simulink model "sim_rx160_two"  (R2020a)
settings: Solver=FixedStepAuto  StartTime=0.0  StopTime=25.0  FixedStep=0.0001  RelTol=1e-3
values from neighbouring files (symbols this model uses):
  cnc_comp = 1    [run_sim_two.m]
  ctc_switch = 0    [run_sim_two.m]
  ctrl_at_end = 1    [run_sim_two.m]
  ctrl_space = 1    [run_sim_two.m]
  ea_set = 4    [run_sim_two.m]
  ea_set2 = 4    [run_sim_two.m]
  ee_att_1 = 3    [run_sim_two.m]
  ee_att_2 = 4    [run_sim_two.m]
  f_des = [0;60;0;0;0;0]    [run_sim_two.m]
  force_ffwd = 1    [run_sim_two.m]
  fp = [p_ef;r_ef]    [run_sim_two.m]
  fp2 = [p_ef2;r_ef2]    [run_sim_two.m]
  frc_comp = 0    [run_sim_two.m]
  grv_comp = 1    [run_sim_two.m]
  ip = [p_ei;r_ei]    [run_sim_two.m]
  ip2 = [p_ei2;r_ei2]    [run_sim_two.m]
  K = 15000    [run_sim_two.m]
  Kc = 0.005    [run_sim_two.m]
  Kd = [10;10;10;7;7;7]    [run_sim_two.m]
  Kdf = [0;10;0;0;0;0]    [run_sim_two.m]
  Ki = [20;20;20;5;5;5]    [run_sim_two.m]
  Kif = [0;0.05;0;0;0;0]    [run_sim_two.m]
  Km = [1;1;1;1;1;1]    [run_sim_two.m]
  Kp = [2550;2250;2750;1150;850;650]    [run_sim_two.m]
  Kpf = [0;3;0;0;0;0]    [run_sim_two.m]
  orn_at_norm = 1    [run_sim_two.m]
  prdc_frc = 0    [run_sim_two.m]
  q_posIni = qi    [run_sim_two.m]
  robot_model_1 = 2    [run_sim_two.m]
  robot_model_2 = 3    [run_sim_two.m]
  rpt_num = 1    [run_sim_two.m]
  rpt_num2 = 10    [run_sim_two.m]
  Sf_diag = [0;1;0;0;0;0]    [run_sim_two.m]
  spr_comp = 1    [run_sim_two.m]
  switch_val = 30    [run_sim_two.m]
  Sx_diag = [1;0;1;1;1;1]    [run_sim_two.m]
  tf2 = rpt_num2 * period2    (= 30)    [run_sim_two.m]
  trj_profile = 3    [run_sim_two.m]
  trj_profile2 = 3    [run_sim_two.m]
  trj_space = 1    [run_sim_two.m]
  trj_space2 = 1    [run_sim_two.m]
  trj_type = 2    [run_sim_two.m]
  trj_type2 = 1    [run_sim_two.m]
undefined symbols (not defined in the file or in its folder): delta
libraries: simulink x2, vrlib x1
(part 1 of 4)
settings Model: Creator=Mertcan  LastModifiedBy=Mertcan

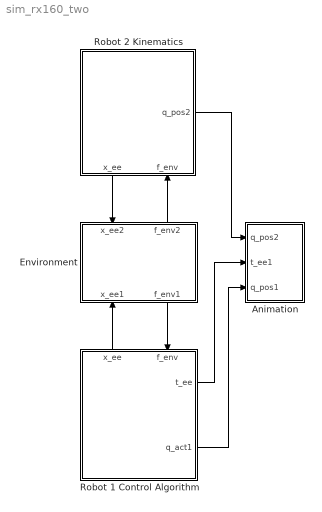
== system sim_rx160_two ==
  Animation : Subsystem
  Environment : Subsystem
      settings: PortSchema="{\"entries\":[{\"content\":{\"sides\":[{\"content\":{\"connectorIds\":[]},\"type\":\"ConnectorPlacement.EquallySpacedRectSide\",\"uuid\":\"b81f9d7c-ea51-4f8c-a6d1-c33009541a36\"},{\"content\":{\"connectorIds\":[],\"side\":\"RIGHT\"},\"type\":\"ConnectorPlacement.EquallySpacedRectSide\",\"uuid\":\"c20f2b2d-2c64-4ed8-b53c-24ad73d5cd54\"},{\"content\":{\"connectorIds\":[\"In1\",\"Out2\"],\"side\":\"TOP\"},\"type\":\"ConnectorPlacement.EquallySpacedRectSide\",\"uuid\":\"f43a164f-97c5-4b00-9b12-265fb19428de\"},{\"content\":{\"connectorIds\":[\"In2\",\"Out1\"],\"side\":\"BOTTOM\"},\"type\":\"ConnectorPlacement.EquallySpacedRectSide\",\"uuid\":\"d7f17a50-52f4-4125-8d61-9ac09671e8dc\"}]},\"type\":\"ConnectorPlacement.EquallySpacedConnector\",\"uuid\":\"950c3a05-8add-442a-8ea6-c018fdaf9f56\"}],\"packageUris\":[\"http://schema.mathworks.com/mf0/Connector/19700101\"],\"version\":\"1.0\"}"
  Robot 1 Control Algorithm : Subsystem
      settings: PortSchema="{\"entries\":[{\"content\":{\"sides\":[{\"content\":{\"connectorIds\":[]},\"type\":\"ConnectorPlacement.EquallySpacedRectSide\",\"uuid\":\"47392d81-5cd8-45f8-ad29-0da949256eb3\"},{\"content\":{\"connectorIds\":[\"Out1\",\"Out2\"],\"side\":\"RIGHT\"},\"type\":\"ConnectorPlacement.EquallySpacedRectSide\",\"uuid\":\"5a0863c0-c1a7-4df3-8221-e3ea3d33c666\"},{\"content\":{\"connectorIds\":[\"Out3\",\"In1\"],\"side\":\"TOP\"},\"type\":\"ConnectorPlacement.EquallySpacedRectSide\",\"uuid\":\"28f918bb-73f1-4e03-a0cb-888dc6781294\"}]},\"type\":\"ConnectorPlacement.EquallySpacedConnector\",\"uuid\":\"b4230a2e-6344-4b3a-b073-8568d43384b7\"}],\"packageUris\":[\"http://schema.mathworks.com/mf0/Connector/19700101\"],\"version\":\"1.0\"}"
  Robot 2 Kinematics : Subsystem
      settings: PortSchema="{\"entries\":[{\"content\":{\"sides\":[{\"content\":{\"connectorIds\":[]},\"type\":\"ConnectorPlacement.EquallySpacedRectSide\",\"uuid\":\"06d4e949-d13f-43fd-bad1-d4926d3f90f8\"},{\"content\":{\"connectorIds\":[\"Out1\"],\"side\":\"RIGHT\"},\"type\":\"ConnectorPlacement.EquallySpacedRectSide\",\"uuid\":\"adb74b17-df4f-4ce7-9c5d-0d46b17775e1\"},{\"content\":{\"connectorIds\":[],\"side\":\"TOP\"},\"type\":\"ConnectorPlacement.EquallySpacedRectSide\",\"uuid\":\"027ceef2-46ca-496b-9cf9-d4a075cf88e8\"},{\"content\":{\"connectorIds\":[\"Out2\",\"In1\"],\"side\":\"BOTTOM\"},\"type\":\"ConnectorPlacement.EquallySpacedRectSide\",\"uuid\":\"2a56aa09-e58e-46c8-9028-b2a4f912dfd9\"}]},\"type\":\"ConnectorPlacement.EquallySpacedConnector\",\"uuid\":\"bb8ed53b-f9bb-471c-90fa-3cf739bcb86a\"}],\"packageUris\":[\"http://schema.mathworks.com/mf0/Connector/19700101\"],\"version\":\"1.0\"}"
  wires:
  Robot 1 Control Algorithm/2(q_act1) -> Animation/3(q_pos1)
  Robot 1 Control Algorithm/3(x_ee) -> Environment/2(x_ee1)
  Robot 2 Kinematics/2(x_ee) -> Environment/1(x_ee2)
  Robot 2 Kinematics/1(q_pos2) -> Animation/1(q_pos2)
  Environment/2(f_env2) -> Robot 2 Kinematics/1(f_env)
  Environment/1(f_env1) -> Robot 1 Control Algorithm/1(f_env)
  Robot 1 Control Algorithm/1(t_ee) -> Animation/2(t_ee1)

== system sim_rx160_two/Animation ==
  q_pos2 : Inport
  t_ee1 : Inport  Port=2
  q_pos1 : Inport  Port=3
  Constant : Constant  Value=1e3
  Demux : Demux  Outputs=2
  Demux1 : Demux  Outputs=2
  Demux2 : Demux  Outputs=3
  Product : Product
  Terminator{,1..3} (4 alike) : Terminator
  To Workspace1 : ToWorkspace  VariableName=eePosCompress  SaveFormat=Timeseries  SampleTime=-1
  VR Sink1 : vrlib/VR Sink  InstantiateOnLoad=on  SampleTime=0.1  ViewEnable=on  RemoteChange=off  RemoteView=off  FieldsWritten=joint_joint_1.rotation.4.1.1.double#joint_joint_2.rotation.4.1.1.double#joint_joint_3.rotation.4.1.1.double#joint_joint_4.rotation.4.1.1.double#joint_joint_5.rotation.4.1.1.double#joint_joint_6.rotation.4.1.1.double#rod_sphere.translation.3.1.1.double#joint_joint_1_0001.rotation.4.1.1.double#joint_joint_2_0001.rotation.4.1.1.double#joint_joint_3_0001.rotation.4.1.1.double#joint_joint_4_0001.rotation.4.1.1.double#joint_joint_5_0001.rotation.4.1.1.double#joint_joint_6_0001.rotation.4.1.1.double  WorldFileName=vr_two_robots_base.x3d  WorldDescription=Dual Robot Scene  AutoView=on  VideoDimensions=[]  AllowVariableSize=off  FigureProperties="{'Position', 'Name', 'Viewpoint', 'CameraBound', 'CameraDirection', 'CameraPosition', 'CameraUpVector', 'ZoomFactor', 'Antialiasing', 'Headlight', 'Lighting', 'NavPanel', 'Sound', 'StatusBar', 'Stereo3D', 'Stereo3DCameraOffset', 'Stereo3DHIT', 'ToolBar', 'Textures', 'Transparency', 'Triad', 'Wireframe', 'NavZones', 'NavMode', 'NavSpeed', 'CaptureFileFormat', 'CaptureFileName', 'Record2DCompressMethod', 'Record2DCompressQuality', 'Record2D', 'Record2DFileName', 'Record2DFPS'; [6.7200000000000000e+02   1.4000000000000000e+02   1.2650000000000000e+03   8.6600000000000000e+02], 'Dual Robot Scene', 'Close View', 'on', [7.6932062354180764e-01  -2.9764832033430183e-01   5.6528864803339762e-01], [-2.2764959269905676e+00   1.1380972332277657e+00  -5.1769680390843549e+00], [2.8408866371190472e-01   9.5192433072198179e-01   1.1460235481843387e-01], [1.0000000000000000e+00], 'on', 'on', 'on', 'halfbar', 'on', 'on', 'off', [1.0000000149011612e-01], [0.0000000000000000e+00], 'on', 'on', 'on', 'none', 'off', 'off', 'examine', 'normal', 'tif', '%f_anim_%n.tif', 'auto', [7.5000000000000000e+01], 'off', '%f_anim_%n.avi', 'auto'}"
  Zero-Order Hold : ZeroOrderHold  SampleTime=0.004
  fwd kin : MATLAB Function  TreatAsAtomicUnit=on
  fwd kin1 : MATLAB Function  TreatAsAtomicUnit=on
  wires:
  q_pos1/1 -> Demux/1
  Demux/1 -> fwd kin/1(u)
  Demux/2 -> Terminator/1
  q_pos2/1 -> Demux1/1
  Demux1/2 -> Terminator1/1
  Demux1/1 -> fwd kin1/1(u)
  fwd kin/1(r1) -> VR Sink1/1
  fwd kin/2(r2) -> VR Sink1/2
  fwd kin/3(r3) -> VR Sink1/3
  fwd kin/4(r4) -> VR Sink1/4
  fwd kin/5(r5) -> VR Sink1/5
  fwd kin/6(r6) -> VR Sink1/6
  fwd kin1/1(r1) -> VR Sink1/8
  fwd kin1/2(r2) -> VR Sink1/9
  fwd kin1/3(r3) -> VR Sink1/10
  fwd kin1/4(r4) -> VR Sink1/11
  fwd kin1/5(r5) -> VR Sink1/12
  fwd kin1/6(r6) -> VR Sink1/13
  t_ee1/1 -> Product/2, Demux2/1
  Product/1 -> VR Sink1/7
  Constant/1 -> Product/1
  Demux2/1 -> Terminator2/1
  Demux2/2 -> Terminator3/1
  Zero-Order Hold/1 -> To Workspace1/1
  Demux2/3 -> Zero-Order Hold/1

== system sim_rx160_two/Environment ==
  x_ee2 : Inport
  x_ee1 : Inport  Port=2
  Clock : Clock  Commented=on
  Constant : Constant  Value=-1
  Constant2 : Constant  Commented=on  Value=[0;0;0]
  MATLAB Function : MATLAB Function  Commented=on  TreatAsAtomicUnit=on
  MATLAB Function1 : MATLAB Function  TreatAsAtomicUnit=on
  MATLAB Function2 : MATLAB Function  Commented=on  TreatAsAtomicUnit=on
  MATLAB Function3 : MATLAB Function  Commented=on  TreatAsAtomicUnit=on
  Product : Product
  Scope : Scope  Commented=on
  Stifness : Constant  Commented=on  Value=K
  Stifness1 : Constant  Value=K
  To Workspace1 : ToWorkspace  Commented=on  VariableName=obsPos  SaveFormat=Timeseries  SampleTime=-1
  delta : Constant  Commented=on  Value=delta
  end-effector attach : Constant  Value=ee_att_1
  f_env1 : Outport
  f_env2 : Outport  Port=2
  wires:
  Stifness/1 -> MATLAB Function/1(K)
  Clock/1 -> MATLAB Function/4(t)
  MATLAB Function/2(x) -> To Workspace1/1, Scope/1
  delta/1 -> MATLAB Function/2(delta)
  x_ee2/1 -> MATLAB Function1/3(x2)
  Product/1 -> f_env2/1
  x_ee1/1 -> MATLAB Function1/1(x1)  "x"
  Stifness1/1 -> MATLAB Function1/4(K)
  MATLAB Function1/1(f_e) -> Product/2, f_env1/1
  Constant2/1 -> MATLAB Function/3(u)
  Constant/1 -> Product/1
  end-effector attach/1 -> MATLAB Function1/2(ee_att_1)

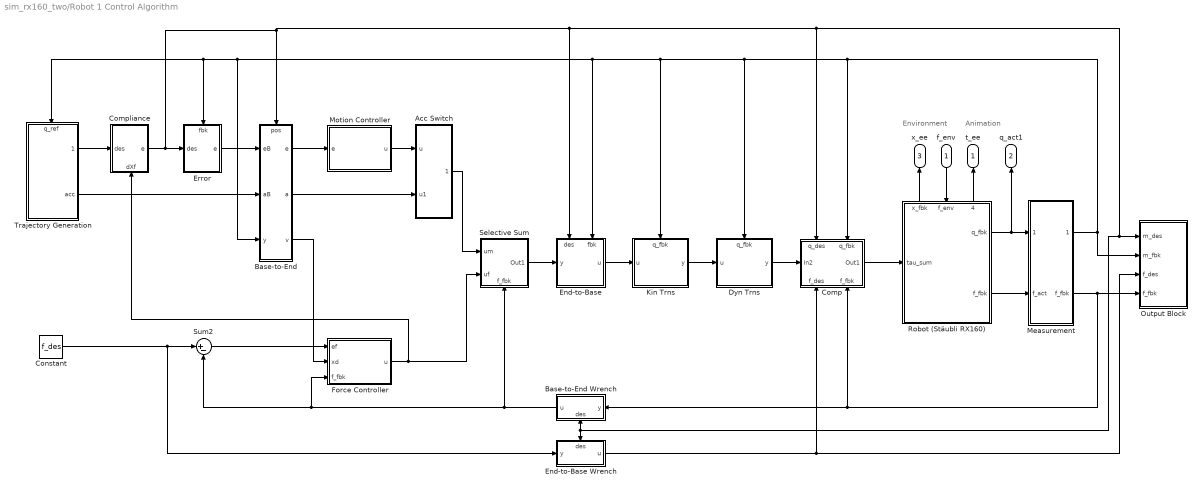
== system sim_rx160_two/Robot 1 Control Algorithm ==
  note: Animation
  note: Environment
  f_env : Inport
  Acc Switch : Subsystem
  Base-to-End : Subsystem
      settings: PortSchema="{\"entries\":[{\"content\":{\"sides\":[{\"content\":{\"connectorIds\":[\"In1\",\"In2\",\"In3\"]},\"type\":\"ConnectorPlacement.EquallySpacedRectSide\",\"uuid\":\"020565b3-ffe2-42af-b350-3d5bbba08d44\"},{\"content\":{\"connectorIds\":[\"Out1\",\"Out2\",\"Out3\"],\"side\":\"RIGHT\"},\"type\":\"ConnectorPlacement.EquallySpacedRectSide\",\"uuid\":\"dbb2181b-8ce7-432e-bb43-e79a64d985e0\"},{\"content\":{\"connectorIds\":[\"In4\"],\"side\":\"TOP\"},\"type\":\"ConnectorPlacement.EquallySpacedRectSide\",\"uuid\":\"edd439a8-cf84-4371-9d31-8030538399a3\"}]},\"type\":\"ConnectorPlacement.EquallySpacedConnector\",\"uuid\":\"06f3d9c3-bbec-4c64-9009-98f920580bff\"}],\"packageUris\":[\"http://schema.mathworks.com/mf0/Connector/19700101\"],\"version\":\"1.0\"}"
  Base-to-End Wrench : Subsystem
      settings: PortSchema="{\"entries\":[{\"content\":{\"sides\":[{\"content\":{\"connectorIds\":[\"In1\"]},\"type\":\"ConnectorPlacement.EquallySpacedRectSide\",\"uuid\":\"020565b3-ffe2-42af-b350-3d5bbba08d44\"},{\"content\":{\"connectorIds\":[\"Out1\"],\"side\":\"RIGHT\"},\"type\":\"ConnectorPlacement.EquallySpacedRectSide\",\"uuid\":\"dbb2181b-8ce7-432e-bb43-e79a64d985e0\"},{\"content\":{\"connectorIds\":[],\"side\":\"TOP\"},\"type\":\"ConnectorPlacement.EquallySpacedRectSide\",\"uuid\":\"edd439a8-cf84-4371-9d31-8030538399a3\"},{\"content\":{\"connectorIds\":[\"In2\"],\"side\":\"BOTTOM\"},\"type\":\"ConnectorPlacement.EquallySpacedRectSide\",\"uuid\":\"efdc06f9-64f5-4bb4-980e-2734ab920eb4\"}]},\"type\":\"ConnectorPlacement.EquallySpacedConnector\",\"uuid\":\"06f3d9c3-bbec-4c64-9009-98f920580bff\"}],\"packageUris\":[\"http://schema.mathworks.com/mf0/Connector/19700101\"],\"version\":\"1.0\"}"
  Comp : Subsystem
      settings: PortSchema="{\"entries\":[{\"content\":{\"sides\":[{\"content\":{\"connectorIds\":[\"In1\"]},\"type\":\"ConnectorPlacement.EquallySpacedRectSide\",\"uuid\":\"b4f3562c-3a59-4f04-a3b3-da66869d7fb8\"},{\"content\":{\"connectorIds\":[\"Out1\"],\"side\":\"RIGHT\"},\"type\":\"ConnectorPlacement.EquallySpacedRectSide\",\"uuid\":\"1269bb29-09be-43cb-9af3-f74a6a005ad0\"},{\"content\":{\"connectorIds\":[\"In2\",\"In3\"],\"side\":\"TOP\"},\"type\":\"ConnectorPlacement.EquallySpacedRectSide\",\"uuid\":\"acd55610-2ecf-4dcc-b0bc-a4343bb42bde\"},{\"content\":{\"connectorIds\":[\"In4\",\"In5\"],\"side\":\"BOTTOM\"},\"type\":\"ConnectorPlacement.EquallySpacedRectSide\",\"uuid\":\"40156ef2-2d75-41dd-a033-e544f1ff9354\"}]},\"type\":\"ConnectorPlacement.EquallySpacedConnector\",\"uuid\":\"953ff7fc-1f3b-47dc-a69f-74118f573792\"}],\"packageUris\":[\"http://schema.mathworks.com/mf0/Connector/19700101\"],\"version\":\"1.0\"}"
  Compliance : Subsystem
      settings: PortSchema="{\"entries\":[{\"content\":{\"sides\":[{\"content\":{\"connectorIds\":[\"In1\"]},\"type\":\"ConnectorPlacement.EquallySpacedRectSide\",\"uuid\":\"178f6af3-2ba7-43c9-b15c-ce5e8339bdff\"},{\"content\":{\"connectorIds\":[\"Out1\"],\"side\":\"RIGHT\"},\"type\":\"ConnectorPlacement.EquallySpacedRectSide\",\"uuid\":\"a6ae646a-c86d-4621-9c36-e111e1f88696\"},{\"content\":{\"connectorIds\":[],\"side\":\"TOP\"},\"type\":\"ConnectorPlacement.EquallySpacedRectSide\",\"uuid\":\"808e2785-04c0-49cf-ade9-42ab28b9e69b\"},{\"content\":{\"connectorIds\":[\"In2\"],\"side\":\"BOTTOM\"},\"type\":\"ConnectorPlacement.EquallySpacedRectSide\",\"uuid\":\"5e5af769-b9d3-4274-a83d-533a837274af\"}]},\"type\":\"ConnectorPlacement.EquallySpacedConnector\",\"uuid\":\"8e74479a-b980-46f8-8664-436c69a1a6e0\"}],\"packageUris\":[\"http://schema.mathworks.com/mf0/Connector/19700101\"],\"version\":\"1.0\"}"
  Constant : Constant  Value=f_des
  Dyn Trns : Subsystem
      settings: PortSchema="{\"entries\":[{\"content\":{\"sides\":[{\"content\":{\"connectorIds\":[\"In1\"]},\"type\":\"ConnectorPlacement.EquallySpacedRectSide\",\"uuid\":\"b813e676-63a5-423f-a8fb-c61aa562c7ca\"},{\"content\":{\"connectorIds\":[\"Out1\"],\"side\":\"RIGHT\"},\"type\":\"ConnectorPlacement.EquallySpacedRectSide\",\"uuid\":\"4be16838-ab6b-4909-a3bd-a94cc7d57bb6\"},{\"content\":{\"connectorIds\":[\"In2\"],\"side\":\"TOP\"},\"type\":\"ConnectorPlacement.EquallySpacedRectSide\",\"uuid\":\"1ff041d7-0766-44e3-aab7-ad2a75321725\"},{\"content\":{\"connectorIds\":[],\"side\":\"BOTTOM\"},\"type\":\"ConnectorPlacement.EquallySpacedRectSide\",\"uuid\":\"f928bd91-1fe8-4da1-ba92-0943790ffd46\"}]},\"type\":\"ConnectorPlacement.EquallySpacedConnector\",\"uuid\":\"28f3288f-f4ad-4a8c-a989-5860322fd42e\"}],\"packageUris\":[\"http://schema.mathworks.com/mf0/Connector/19700101\"],\"version\":\"1.0\"}"
  End-to-Base : Subsystem
      settings: PortSchema="{\"entries\":[{\"content\":{\"sides\":[{\"content\":{\"connectorIds\":[\"In1\"]},\"type\":\"ConnectorPlacement.EquallySpacedRectSide\",\"uuid\":\"020565b3-ffe2-42af-b350-3d5bbba08d44\"},{\"content\":{\"connectorIds\":[\"Out1\"],\"side\":\"RIGHT\"},\"type\":\"ConnectorPlacement.EquallySpacedRectSide\",\"uuid\":\"dbb2181b-8ce7-432e-bb43-e79a64d985e0\"},{\"content\":{\"connectorIds\":[\"In2\",\"In3\"],\"side\":\"TOP\"},\"type\":\"ConnectorPlacement.EquallySpacedRectSide\",\"uuid\":\"edd439a8-cf84-4371-9d31-8030538399a3\"}]},\"type\":\"ConnectorPlacement.EquallySpacedConnector\",\"uuid\":\"06f3d9c3-bbec-4c64-9009-98f920580bff\"}],\"packageUris\":[\"http://schema.mathworks.com/mf0/Connector/19700101\"],\"version\":\"1.0\"}"
  End-to-Base Wrench : Subsystem
      settings: PortSchema="{\"entries\":[{\"content\":{\"sides\":[{\"content\":{\"connectorIds\":[\"In1\"]},\"type\":\"ConnectorPlacement.EquallySpacedRectSide\",\"uuid\":\"020565b3-ffe2-42af-b350-3d5bbba08d44\"},{\"content\":{\"connectorIds\":[\"Out1\"],\"side\":\"RIGHT\"},\"type\":\"ConnectorPlacement.EquallySpacedRectSide\",\"uuid\":\"dbb2181b-8ce7-432e-bb43-e79a64d985e0\"},{\"content\":{\"connectorIds\":[\"In2\"],\"side\":\"TOP\"},\"type\":\"ConnectorPlacement.EquallySpacedRectSide\",\"uuid\":\"edd439a8-cf84-4371-9d31-8030538399a3\"}]},\"type\":\"ConnectorPlacement.EquallySpacedConnector\",\"uuid\":\"06f3d9c3-bbec-4c64-9009-98f920580bff\"}],\"packageUris\":[\"http://schema.mathworks.com/mf0/Connector/19700101\"],\"version\":\"1.0\"}"
  Error : Subsystem
      settings: PortSchema="{\"entries\":[{\"content\":{\"sides\":[{\"content\":{\"connectorIds\":[\"In1\"]},\"type\":\"ConnectorPlacement.EquallySpacedRectSide\",\"uuid\":\"178f6af3-2ba7-43c9-b15c-ce5e8339bdff\"},{\"content\":{\"connectorIds\":[\"Out1\"],\"side\":\"RIGHT\"},\"type\":\"ConnectorPlacement.EquallySpacedRectSide\",\"uuid\":\"a6ae646a-c86d-4621-9c36-e111e1f88696\"},{\"content\":{\"connectorIds\":[\"In2\"],\"side\":\"TOP\"},\"type\":\"ConnectorPlacement.EquallySpacedRectSide\",\"uuid\":\"808e2785-04c0-49cf-ade9-42ab28b9e69b\"},{\"content\":{\"connectorIds\":[],\"side\":\"BOTTOM\"},\"type\":\"ConnectorPlacement.EquallySpacedRectSide\",\"uuid\":\"5e5af769-b9d3-4274-a83d-533a837274af\"}]},\"type\":\"ConnectorPlacement.EquallySpacedConnector\",\"uuid\":\"8e74479a-b980-46f8-8664-436c69a1a6e0\"}],\"packageUris\":[\"http://schema.mathworks.com/mf0/Connector/19700101\"],\"version\":\"1.0\"}"
  Force Controller : Subsystem
  Kin Trns : Subsystem
      settings: PortSchema="{\"entries\":[{\"content\":{\"sides\":[{\"content\":{\"connectorIds\":[\"In1\"]},\"type\":\"ConnectorPlacement.EquallySpacedRectSide\",\"uuid\":\"178f6af3-2ba7-43c9-b15c-ce5e8339bdff\"},{\"content\":{\"connectorIds\":[\"Out1\"],\"side\":\"RIGHT\"},\"type\":\"ConnectorPlacement.EquallySpacedRectSide\",\"uuid\":\"a6ae646a-c86d-4621-9c36-e111e1f88696\"},{\"content\":{\"connectorIds\":[\"In2\"],\"side\":\"TOP\"},\"type\":\"ConnectorPlacement.EquallySpacedRectSide\",\"uuid\":\"808e2785-04c0-49cf-ade9-42ab28b9e69b\"},{\"content\":{\"connectorIds\":[],\"side\":\"BOTTOM\"},\"type\":\"ConnectorPlacement.EquallySpacedRectSide\",\"uuid\":\"859c665c-c9df-42d0-801f-28168852978e\"}]},\"type\":\"ConnectorPlacement.EquallySpacedConnector\",\"uuid\":\"8e74479a-b980-46f8-8664-436c69a1a6e0\"}],\"packageUris\":[\"http://schema.mathworks.com/mf0/Connector/19700101\"],\"version\":\"1.0\"}"
  Measurement : Subsystem
  Motion Controller : Subsystem
  Output Block : Subsystem
  Robot (Stäubli RX160) : Subsystem
      settings: PortSchema="{\"entries\":[{\"content\":{\"sides\":[{\"content\":{\"connectorIds\":[\"In1\"]},\"type\":\"ConnectorPlacement.EquallySpacedRectSide\",\"uuid\":\"6284adc3-d758-45ef-9141-dee680c83b08\"},{\"content\":{\"connectorIds\":[\"Out1\",\"Out2\"],\"side\":\"RIGHT\"},\"type\":\"ConnectorPlacement.EquallySpacedRectSide\",\"uuid\":\"181d7ec4-49ad-445a-9254-c2b56cfcaf16\"},{\"content\":{\"connectorIds\":[\"Out3\",\"In2\",\"Out4\"],\"side\":\"TOP\"},\"type\":\"ConnectorPlacement.EquallySpacedRectSide\",\"uuid\":\"b714267f-2932-4320-9de1-3f424c8ad2a6\"}]},\"type\":\"ConnectorPlacement.EquallySpacedConnector\",\"uuid\":\"69d7b4c6-737c-4cfe-af82-254ae10a5bd4\"}],\"packageUris\":[\"http://schema.mathworks.com/mf0/Connector/19700101\"],\"version\":\"1.0\"}"
      mask Display: image('$imagefile'); % Use "Edit Image" on toolstrip to change.
  Selective Sum : Subsystem
      settings: PortSchema="{\"entries\":[{\"content\":{\"sides\":[{\"content\":{\"connectorIds\":[\"In1\",\"In2\"]},\"type\":\"ConnectorPlacement.EquallySpacedRectSide\",\"uuid\":\"dbbbc107-fbc8-47f5-9d95-7600de16627b\"},{\"content\":{\"connectorIds\":[\"Out1\"],\"side\":\"RIGHT\"},\"type\":\"ConnectorPlacement.EquallySpacedRectSide\",\"uuid\":\"8787e853-c330-4d61-8f58-c17085830519\"},{\"content\":{\"connectorIds\":[],\"side\":\"TOP\"},\"type\":\"ConnectorPlacement.EquallySpacedRectSide\",\"uuid\":\"f03d7db1-6e8a-4daf-a27a-f65505c3a089\"},{\"content\":{\"connectorIds\":[\"In3\"],\"side\":\"BOTTOM\"},\"type\":\"ConnectorPlacement.EquallySpacedRectSide\",\"uuid\":\"fa988798-1e34-4fa1-8ebc-2815db113161\"}]},\"type\":\"ConnectorPlacement.EquallySpacedConnector\",\"uuid\":\"12668bfd-1d91-401f-8203-13ab9cac1f2c\"}],\"packageUris\":[\"http://schema.mathworks.com/mf0/Connector/19700101\"],\"version\":\"1.0\"}"
  Sum2 : Sum  Inputs=|+-
  Trajectory Generation : Subsystem
      settings: PortSchema="{\"entries\":[{\"content\":{\"sides\":[{\"content\":{\"connectorIds\":[]},\"type\":\"ConnectorPlacement.EquallySpacedRectSide\",\"uuid\":\"4512f7c1-141f-4ca9-8985-d7b3fc7dc203\"},{\"content\":{\"connectorIds\":[\"Out1\",\"Out2\"],\"side\":\"RIGHT\"},\"type\":\"ConnectorPlacement.EquallySpacedRectSide\",\"uuid\":\"5c5a9662-9ae9-4eb5-828e-be3fe6f4b168\"},{\"content\":{\"connectorIds\":[\"In1\"],\"side\":\"TOP\"},\"type\":\"ConnectorPlacement.EquallySpacedRectSide\",\"uuid\":\"4c26be9f-0fe4-4a1d-a76a-786ec65b737d\"},{\"content\":{\"connectorIds\":[],\"side\":\"BOTTOM\"},\"type\":\"ConnectorPlacement.EquallySpacedRectSide\",\"uuid\":\"9d756de9-72bc-4633-ac1d-40b2671d614a\"}]},\"type\":\"ConnectorPlacement.EquallySpacedConnector\",\"uuid\":\"303d3c57-cadd-4518-8f0b-ca4d9a4186ef\"}],\"packageUris\":[\"http://schema.mathworks.com/mf0/Connector/19700101\"],\"version\":\"1.0\"}"
  t_ee : Outport
  q_act1 : Outport  Port=2
  x_ee : Outport  Port=3
  wires:
  Robot (Stäubli RX160)/1(q_fbk) -> Measurement/1(q_act), q_act1/1
  Constant/1 -> End-to-Base Wrench/1(y), Sum2/1
  Robot (Stäubli RX160)/2(f_fbk) -> Measurement/2(f_act)
  Acc Switch/1(Out1) -> Selective Sum/1(um)
  Comp/1(Out1) -> Robot (Stäubli RX160)/1(tau_sum)
  Measurement/2(f_fbk) -> Comp/5(f_fbk), Base-to-End Wrench/1(y), Output Block/4(f_fbk)
  Dyn Trns/1(y) -> Comp/1(In2)
  Trajectory Generation/2(acc) -> Base-to-End/2(aB)
  Robot (Stäubli RX160)/3(x_fbk) -> x_ee/1
  Kin Trns/1(y) -> Dyn Trns/1(u)
  f_env/1 -> Robot (Stäubli RX160)/2(f_env)
  Motion Controller/1(u) -> Acc Switch/1(u)
  Sum2/1 -> Force Controller/1(ef)
  Robot (Stäubli RX160)/4(x_compress) -> t_ee/1
  Selective Sum/1(Out1) -> End-to-Base/1(y)
  End-to-Base/1(u) -> Kin Trns/1(u)
  Error/1(e) -> Base-to-End/1(eB)
  Base-to-End/1(e) -> Motion Controller/1(e)
  Base-to-End/3(v) -> Force Controller/2(xd)
  Measurement/1(m_fbk) -> Output Block/2(m_fbk), Comp/3(q_fbk), Dyn Trns/2(q_fbk), End-to-Base/3(fbk), Base-to-End/3(y), Error/2(fbk), Trajectory Generation/1(q_ref), Kin Trns/2(q_fbk)
  Base-to-End/2(a) -> Acc Switch/2(u1)
  End-to-Base Wrench/1(u) -> Output Block/3(f_des), Comp/4(f_des)
  Base-to-End Wrench/1(u) -> Selective Sum/3(f_fbk), Force Controller/3(f_fbk), Sum2/2
  Force Controller/1(u) -> Compliance/2(dXf), Selective Sum/2(uf)
  Compliance/1(e) -> Comp/2(q_des), Output Block/1(m_des), End-to-Base Wrench/2(des), Base-to-End Wrench/2(des), End-to-Base/2(des), Base-to-End/4(pos), Error/1(des)
  Trajectory Generation/1(pos&vel) -> Compliance/1(des)

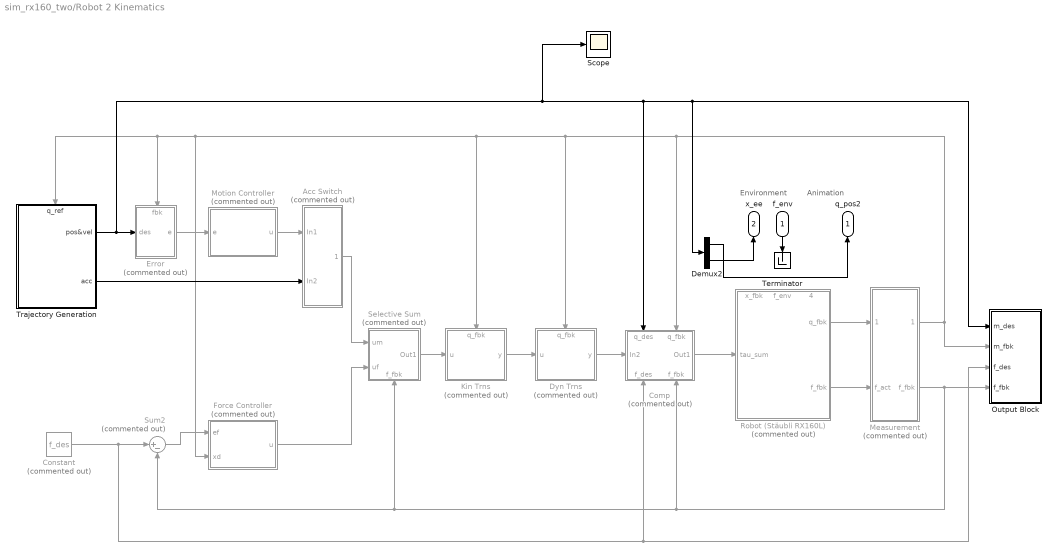
== system sim_rx160_two/Robot 2 Kinematics ==
  note: Animation
  note: Environment
  f_env : Inport  PortDimensions=6
  Acc Switch : Subsystem  Commented=on
  Comp : Subsystem  Commented=on
      settings: PortSchema="{\"entries\":[{\"content\":{\"sides\":[{\"content\":{\"connectorIds\":[\"In1\"]},\"type\":\"ConnectorPlacement.EquallySpacedRectSide\",\"uuid\":\"b4f3562c-3a59-4f04-a3b3-da66869d7fb8\"},{\"content\":{\"connectorIds\":[\"Out1\"],\"side\":\"RIGHT\"},\"type\":\"ConnectorPlacement.EquallySpacedRectSide\",\"uuid\":\"1269bb29-09be-43cb-9af3-f74a6a005ad0\"},{\"content\":{\"connectorIds\":[\"In2\",\"In3\"],\"side\":\"TOP\"},\"type\":\"ConnectorPlacement.EquallySpacedRectSide\",\"uuid\":\"acd55610-2ecf-4dcc-b0bc-a4343bb42bde\"},{\"content\":{\"connectorIds\":[\"In4\",\"In5\"],\"side\":\"BOTTOM\"},\"type\":\"ConnectorPlacement.EquallySpacedRectSide\",\"uuid\":\"40156ef2-2d75-41dd-a033-e544f1ff9354\"}]},\"type\":\"ConnectorPlacement.EquallySpacedConnector\",\"uuid\":\"953ff7fc-1f3b-47dc-a69f-74118f573792\"}],\"packageUris\":[\"http://schema.mathworks.com/mf0/Connector/19700101\"],\"version\":\"1.0\"}"
  Constant : Constant  Commented=on  Value=f_des
  Demux2 : Demux  Outputs=[12;18]
  Dyn Trns : Subsystem  Commented=on
      settings: PortSchema="{\"entries\":[{\"content\":{\"sides\":[{\"content\":{\"connectorIds\":[\"In1\"]},\"type\":\"ConnectorPlacement.EquallySpacedRectSide\",\"uuid\":\"b813e676-63a5-423f-a8fb-c61aa562c7ca\"},{\"content\":{\"connectorIds\":[\"Out1\"],\"side\":\"RIGHT\"},\"type\":\"ConnectorPlacement.EquallySpacedRectSide\",\"uuid\":\"4be16838-ab6b-4909-a3bd-a94cc7d57bb6\"},{\"content\":{\"connectorIds\":[\"In2\"],\"side\":\"TOP\"},\"type\":\"ConnectorPlacement.EquallySpacedRectSide\",\"uuid\":\"1ff041d7-0766-44e3-aab7-ad2a75321725\"},{\"content\":{\"connectorIds\":[],\"side\":\"BOTTOM\"},\"type\":\"ConnectorPlacement.EquallySpacedRectSide\",\"uuid\":\"f928bd91-1fe8-4da1-ba92-0943790ffd46\"}]},\"type\":\"ConnectorPlacement.EquallySpacedConnector\",\"uuid\":\"28f3288f-f4ad-4a8c-a989-5860322fd42e\"}],\"packageUris\":[\"http://schema.mathworks.com/mf0/Connector/19700101\"],\"version\":\"1.0\"}"
  Error : Subsystem  Commented=on
      settings: PortSchema="{\"entries\":[{\"content\":{\"sides\":[{\"content\":{\"connectorIds\":[\"In1\"]},\"type\":\"ConnectorPlacement.EquallySpacedRectSide\",\"uuid\":\"178f6af3-2ba7-43c9-b15c-ce5e8339bdff\"},{\"content\":{\"connectorIds\":[\"Out1\"],\"side\":\"RIGHT\"},\"type\":\"ConnectorPlacement.EquallySpacedRectSide\",\"uuid\":\"a6ae646a-c86d-4621-9c36-e111e1f88696\"},{\"content\":{\"connectorIds\":[\"In2\"],\"side\":\"TOP\"},\"type\":\"ConnectorPlacement.EquallySpacedRectSide\",\"uuid\":\"808e2785-04c0-49cf-ade9-42ab28b9e69b\"},{\"content\":{\"connectorIds\":[],\"side\":\"BOTTOM\"},\"type\":\"ConnectorPlacement.EquallySpacedRectSide\",\"uuid\":\"5e5af769-b9d3-4274-a83d-533a837274af\"}]},\"type\":\"ConnectorPlacement.EquallySpacedConnector\",\"uuid\":\"8e74479a-b980-46f8-8664-436c69a1a6e0\"}],\"packageUris\":[\"http://schema.mathworks.com/mf0/Connector/19700101\"],\"version\":\"1.0\"}"
  Force Controller : Subsystem  Commented=on
  Kin Trns : Subsystem  Commented=on
      settings: PortSchema="{\"entries\":[{\"content\":{\"sides\":[{\"content\":{\"connectorIds\":[\"In1\"]},\"type\":\"ConnectorPlacement.EquallySpacedRectSide\",\"uuid\":\"178f6af3-2ba7-43c9-b15c-ce5e8339bdff\"},{\"content\":{\"connectorIds\":[\"Out1\"],\"side\":\"RIGHT\"},\"type\":\"ConnectorPlacement.EquallySpacedRectSide\",\"uuid\":\"a6ae646a-c86d-4621-9c36-e111e1f88696\"},{\"content\":{\"connectorIds\":[\"In2\"],\"side\":\"TOP\"},\"type\":\"ConnectorPlacement.EquallySpacedRectSide\",\"uuid\":\"808e2785-04c0-49cf-ade9-42ab28b9e69b\"},{\"content\":{\"connectorIds\":[],\"side\":\"BOTTOM\"},\"type\":\"ConnectorPlacement.EquallySpacedRectSide\",\"uuid\":\"859c665c-c9df-42d0-801f-28168852978e\"}]},\"type\":\"ConnectorPlacement.EquallySpacedConnector\",\"uuid\":\"8e74479a-b980-46f8-8664-436c69a1a6e0\"}],\"packageUris\":[\"http://schema.mathworks.com/mf0/Connector/19700101\"],\"version\":\"1.0\"}"
  Measurement : Subsystem  Commented=on
  Motion Controller : Subsystem  Commented=on
  Output Block : Subsystem
  Robot (Stäubli RX160L) : Subsystem  Commented=on
      settings: PortSchema="{\"entries\":[{\"content\":{\"sides\":[{\"content\":{\"connectorIds\":[\"In1\"]},\"type\":\"ConnectorPlacement.EquallySpacedRectSide\",\"uuid\":\"6284adc3-d758-45ef-9141-dee680c83b08\"},{\"content\":{\"connectorIds\":[\"Out1\",\"Out2\"],\"side\":\"RIGHT\"},\"type\":\"ConnectorPlacement.EquallySpacedRectSide\",\"uuid\":\"181d7ec4-49ad-445a-9254-c2b56cfcaf16\"},{\"content\":{\"connectorIds\":[\"Out3\",\"In2\",\"Out4\"],\"side\":\"TOP\"},\"type\":\"ConnectorPlacement.EquallySpacedRectSide\",\"uuid\":\"b714267f-2932-4320-9de1-3f424c8ad2a6\"}]},\"type\":\"ConnectorPlacement.EquallySpacedConnector\",\"uuid\":\"69d7b4c6-737c-4cfe-af82-254ae10a5bd4\"}],\"packageUris\":[\"http://schema.mathworks.com/mf0/Connector/19700101\"],\"version\":\"1.0\"}"
      mask Display: image('$imagefile'); % Use "Edit Image" on toolstrip to change.
  Scope : Scope
  Selective Sum : Subsystem  Commented=on
      settings: PortSchema="{\"entries\":[{\"content\":{\"sides\":[{\"content\":{\"connectorIds\":[\"In1\",\"In2\"]},\"type\":\"ConnectorPlacement.EquallySpacedRectSide\",\"uuid\":\"dbbbc107-fbc8-47f5-9d95-7600de16627b\"},{\"content\":{\"connectorIds\":[\"Out1\"],\"side\":\"RIGHT\"},\"type\":\"ConnectorPlacement.EquallySpacedRectSide\",\"uuid\":\"8787e853-c330-4d61-8f58-c17085830519\"},{\"content\":{\"connectorIds\":[],\"side\":\"TOP\"},\"type\":\"ConnectorPlacement.EquallySpacedRectSide\",\"uuid\":\"f03d7db1-6e8a-4daf-a27a-f65505c3a089\"},{\"content\":{\"connectorIds\":[\"In3\"],\"side\":\"BOTTOM\"},\"type\":\"ConnectorPlacement.EquallySpacedRectSide\",\"uuid\":\"fa988798-1e34-4fa1-8ebc-2815db113161\"}]},\"type\":\"ConnectorPlacement.EquallySpacedConnector\",\"uuid\":\"12668bfd-1d91-401f-8203-13ab9cac1f2c\"}],\"packageUris\":[\"http://schema.mathworks.com/mf0/Connector/19700101\"],\"version\":\"1.0\"}"
  Sum2 : Sum  Commented=on  Inputs=|+-
  Terminator : Terminator
  Trajectory Generation : Subsystem
      settings: PortSchema="{\"entries\":[{\"content\":{\"sides\":[{\"content\":{\"connectorIds\":[]},\"type\":\"ConnectorPlacement.EquallySpacedRectSide\",\"uuid\":\"4512f7c1-141f-4ca9-8985-d7b3fc7dc203\"},{\"content\":{\"connectorIds\":[\"Out1\",\"Out2\"],\"side\":\"RIGHT\"},\"type\":\"ConnectorPlacement.EquallySpacedRectSide\",\"uuid\":\"5c5a9662-9ae9-4eb5-828e-be3fe6f4b168\"},{\"content\":{\"connectorIds\":[\"In1\"],\"side\":\"TOP\"},\"type\":\"ConnectorPlacement.EquallySpacedRectSide\",\"uuid\":\"4c26be9f-0fe4-4a1d-a76a-786ec65b737d\"},{\"content\":{\"connectorIds\":[],\"side\":\"BOTTOM\"},\"type\":\"ConnectorPlacement.EquallySpacedRectSide\",\"uuid\":\"9d756de9-72bc-4633-ac1d-40b2671d614a\"}]},\"type\":\"ConnectorPlacement.EquallySpacedConnector\",\"uuid\":\"303d3c57-cadd-4518-8f0b-ca4d9a4186ef\"}],\"packageUris\":[\"http://schema.mathworks.com/mf0/Connector/19700101\"],\"version\":\"1.0\"}"
  q_pos2 : Outport  PortDimensions=12
  x_ee : Outport  Port=2
  wires:
  Force Controller/1(u) -> Selective Sum/2(uf)
  Motion Controller/1(u) -> Acc Switch/1(In1)
  Measurement/1(m_fbk) -> Output Block/2(m_fbk), Comp/3(q_fbk), Dyn Trns/2(q_fbk), Force Controller/2(xd), Error/2(fbk), Trajectory Generation/1(q_ref), Kin Trns/2(q_fbk)
  Error/1(e) -> Motion Controller/1(e)
  Comp/1(Out1) -> Robot (Stäubli RX160L)/1(tau_sum)
  Acc Switch/1(Out1) -> Selective Sum/1(um)
  Selective Sum/1(Out1) -> Kin Trns/1(u)
  Trajectory Generation/2(acc) -> Acc Switch/2(In2)
  Sum2/1 -> Force Controller/1(ef)
  Robot (Stäubli RX160L)/1(q_fbk) -> Measurement/1(q_act)
  Constant/1 -> Comp/4(f_des), Output Block/3(f_des), Sum2/1
  Robot (Stäubli RX160L)/2(f_fbk) -> Measurement/2(f_act)
  Measurement/2(f_fbk) -> Sum2/2, Selective Sum/3(f_fbk), Comp/5(f_fbk), Output Block/4(f_fbk)
  Dyn Trns/1(y) -> Comp/1(In2)
  Kin Trns/1(y) -> Dyn Trns/1(u)
  Demux2/1 -> q_pos2/1
  Demux2/2 -> x_ee/1
  f_env/1 -> Terminator/1
  Trajectory Generation/1(pos&vel) -> Scope/1, Comp/2(q_des), Output Block/1(m_des), Demux2/1, Error/1(des)

== system sim_rx160_two/Robot 1 Control Algorithm/Acc Switch ==
  u : Inport  PortDimensions=6
  u1 : Inport  Port=2  PortDimensions=6
  Sum : Sum  Inputs=++|
  Switch : Switch  Criteria=u2 > Threshold
  computed torque switch : Constant  Value=ctc_switch
  Out1 : Outport  PortDimensions=6
  wires:
  Sum/1 -> Switch/1
  computed torque switch/1 -> Switch/2
  Switch/1 -> Out1/1
  u/1 -> Switch/3, Sum/1
  u1/1 -> Sum/2

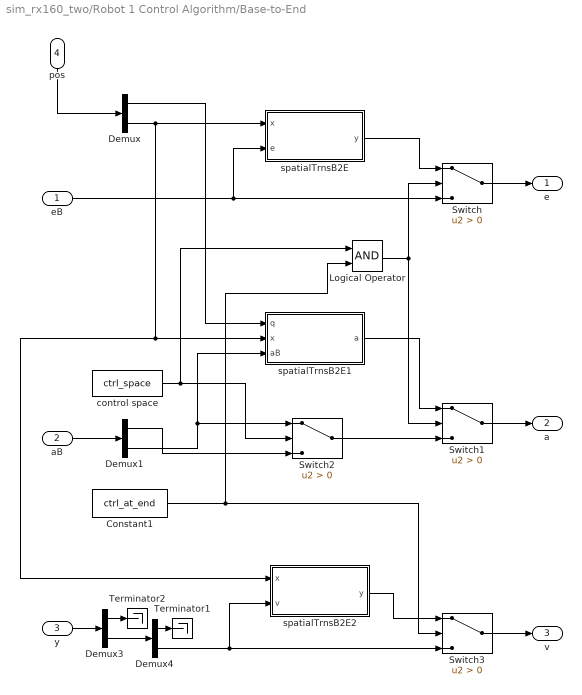
== system sim_rx160_two/Robot 1 Control Algorithm/Base-to-End ==
  eB : Inport  PortDimensions=12
  aB : Inport  Port=2  PortDimensions=12
  y : Inport  Port=3  PortDimensions=30
  pos : Inport  Port=4  PortDimensions=30
  Constant1 : Constant  Value=ctrl_at_end
  Demux : Demux  Outputs=[12;18]
  Demux1 : Demux  Outputs=2
  Demux3 : Demux  Outputs=[12;18]
  Demux4 : Demux  Outputs=[12;6]
  Logical Operator : Logic  AllPortsSameDT=off  OutDataTypeStr=boolean
  Switch{,1..3} (4 alike) : Switch  Criteria=u2 > Threshold
  Terminator1 : Terminator
  Terminator2 : Terminator
  control space : Constant  Value=ctrl_space
  spatialTrnsB2E : MATLAB Function  TreatAsAtomicUnit=on
  spatialTrnsB2E1 : MATLAB Function  TreatAsAtomicUnit=on
  spatialTrnsB2E2 : MATLAB Function  TreatAsAtomicUnit=on
  e : Outport  PortDimensions=12
  a : Outport  Port=2  PortDimensions=6
  v : Outport  Port=3  PortDimensions=6
  wires:
  spatialTrnsB2E/1(y) -> Switch/1
  Demux/1 -> spatialTrnsB2E1/1(q)
  pos/1 -> Demux/1
  eB/1 -> Switch/3, spatialTrnsB2E/2(e)
  Switch/1 -> e/1
  Switch1/1 -> a/1
  spatialTrnsB2E1/1(a) -> Switch1/1
  Logical Operator/1 -> Switch1/2, Switch/2
  control space/1 -> Logical Operator/1, Switch2/2
  aB/1 -> Demux1/1
  Demux1/2 -> Switch2/1, spatialTrnsB2E1/3(aB)
  Switch2/1 -> Switch1/3
  Demux1/1 -> Switch2/3
  Demux3/1 -> Terminator2/1
  y/1 -> Demux3/1
  Demux/2 -> spatialTrnsB2E1/2(x), spatialTrnsB2E2/1(x), spatialTrnsB2E/1(x)
  Demux4/1 -> Terminator1/1
  Demux3/2 -> Demux4/1
  Switch3/1 -> v/1
  spatialTrnsB2E2/1(y) -> Switch3/1
  Demux4/2 -> spatialTrnsB2E2/2(v), Switch3/3
  Constant1/1 -> Logical Operator/2, Switch3/2

== system sim_rx160_two/Robot 1 Control Algorithm/Base-to-End Wrench ==
  y : Inport  PortDimensions=6
  des : Inport  Port=2  PortDimensions=30
  Constant2 : Constant  Value=ctrl_at_end
  Demux : Demux  Outputs=[12;18]
  Switch : Switch  Criteria=u2 > Threshold
  Terminator : Terminator
  f_fbk scope : Scope
  spatialTrnsB2E : MATLAB Function  TreatAsAtomicUnit=on
  u : Outport  PortDimensions=6
  wires:
  y/1 -> Switch/3, spatialTrnsB2E/2(f_fbk)
  spatialTrnsB2E/1(f_fbkE) -> Switch/1
  Constant2/1 -> Switch/2
  des/1 -> Demux/1
  Demux/2 -> spatialTrnsB2E/1(x)
  Demux/1 -> Terminator/1
  Switch/1 -> f_fbk scope/1, u/1

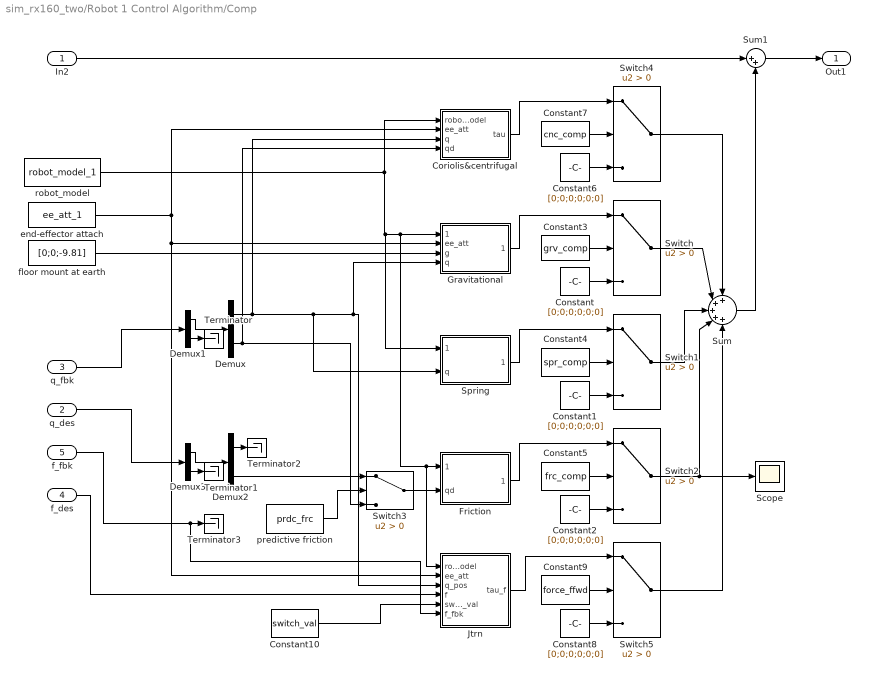
== system sim_rx160_two/Robot 1 Control Algorithm/Comp ==
  In2 : Inport  PortDimensions=6
  q_des : Inport  Port=2  PortDimensions=30
  q_fbk : Inport  Port=3  PortDimensions=30
  f_des : Inport  Port=4  PortDimensions=6
  f_fbk : Inport  Port=5  PortDimensions=6
  Constant{,1..2,6,8} (5 alike) : Constant  Value=[0;0;0;0;0;0]
  Constant10 : Constant  Value=switch_val
  Constant3 : Constant  Value=grv_comp
  Constant4 : Constant  Value=spr_comp
  Constant5 : Constant  Value=frc_comp
  Constant7 : Constant  Value=cnc_comp
  Constant9 : Constant  Value=force_ffwd
  Coriolis&centrifugal : MATLAB Function  TreatAsAtomicUnit=on
  Demux : Demux  Outputs=2
  Demux1 : Demux  Outputs=[12;18]
  Demux2 : Demux  Outputs=2
  Demux3 : Demux  Outputs=[12;18]
  Friction : MATLAB Function  TreatAsAtomicUnit=on
  Gravitational : MATLAB Function  TreatAsAtomicUnit=on
  Jtrn : MATLAB Function  TreatAsAtomicUnit=on
  Scope : Scope
  Spring : MATLAB Function  TreatAsAtomicUnit=on
  Sum : Sum  Inputs=+++++
  Sum1 : Sum  Inputs=|++
  Switch{,1..5} (6 alike) : Switch  Criteria=u2 > Threshold
  Terminator{,1..3} (4 alike) : Terminator
  end-effector attach : Constant  Value=ee_att_1
  floor mount at earth : Constant  Value=[0;0;-9.81]
  predictive friction : Constant  Value=prdc_frc
  robot_model : Constant  Value=robot_model_1
  Out1 : Outport  PortDimensions=6
  wires:
  Sum/1 -> Sum1/2
  Sum1/1 -> Out1/1
  In2/1 -> Sum1/1
  Constant7/1 -> Switch4/2
  Switch1/1 -> Sum/3
  Coriolis&centrifugal/1(tau) -> Switch4/1
  Switch4/1 -> Sum/1
  Demux2/2 -> Switch3/1
  f_fbk/1 -> Jtrn/6(f_fbk), Terminator3/1
  Constant6/1 -> Switch4/3
  q_des/1 -> Demux3/1
  Demux2/1 -> Terminator2/1
  Constant/1 -> Switch/3
  Demux3/2 -> Terminator1/1
  Demux1/1 -> Demux/1
  Constant5/1 -> Switch2/2
  predictive friction/1 -> Switch3/2
  Constant4/1 -> Switch1/2
  Switch/1 -> Sum/2
  robot_model/1 -> Coriolis&centrifugal/1(robot_model), Jtrn/1(robot_model), Friction/1(robot_model), Gravitational/1(robot_model), Spring/1(robot_model)
  q_fbk/1 -> Demux1/1
  Demux3/1 -> Demux2/1
  Spring/1(tau_spr) -> Switch1/1
  Switch2/1 -> Scope/1, Sum/4
  Constant1/1 -> Switch1/3
  Demux/1 -> Jtrn/3(q_pos), Gravitational/4(q), Spring/2(q), Coriolis&centrifugal/3(q)
  Friction/1(tau_frc) -> Switch2/1
  Gravitational/1(tau_grv) -> Switch/1
  Demux1/2 -> Terminator/1
  Demux/2 -> Coriolis&centrifugal/4(qd), Switch3/3
  Constant3/1 -> Switch/2
  Constant2/1 -> Switch2/3
  Switch3/1 -> Friction/2(qd)
  Constant8/1 -> Switch5/3
  Constant9/1 -> Switch5/2
  Jtrn/1(tau_f) -> Switch5/1
  Switch5/1 -> Sum/5
  floor mount at earth/1 -> Gravitational/3(g)
  end-effector attach/1 -> Jtrn/2(ee_att), Gravitational/2(ee_att), Coriolis&centrifugal/2(ee_att)
  f_des/1 -> Jtrn/4(f)
  Constant10/1 -> Jtrn/5(switch_val)

== system sim_rx160_two/Robot 1 Control Algorithm/Compliance ==
  des : Inport  PortDimensions=30
  dXf : Inport  Port=2  PortDimensions=6
  Compliance gain : Constant  Value=Kc
  Integrator : Integrator
  MATLAB Function : MATLAB Function  TreatAsAtomicUnit=on
  Subsystem : Subsystem  Commented=on
  Switch : Switch  Criteria=u2 > Threshold
  Zero-Order Hold : ZeroOrderHold  SampleTime=0.004
  control_space : Constant  Value=orn_at_norm
  e : Outport  PortDimensions=30
  wires:
  control_space/1 -> Switch/2
  MATLAB Function/1(y) -> Zero-Order Hold/1
  Switch/1 -> e/1
  des/1 -> Switch/3, MATLAB Function/1(des)
  dXf/1 -> Integrator/1
  Zero-Order Hold/1 -> Switch/1
  Compliance gain/1 -> MATLAB Function/2(Kc)
  Integrator/1 -> MATLAB Function/3(dXf)

== system sim_rx160_two/Robot 1 Control Algorithm/Dyn Trns ==
  u : Inport
  q_fbk : Inport  Port=2
  Demux : Demux  Outputs=[6;6]
  Demux1 : Demux  Outputs=[12;18]
  MATLAB Function : MATLAB Function  TreatAsAtomicUnit=on
  Switch : Switch  Criteria=u2 > Threshold
  Terminator : Terminator
  Terminator1 : Terminator
  computed torque switch : Constant  Value=ctc_switch
  end-effector attach : Constant  Value=ee_att_1
  robot_model : Constant  Value=robot_model_1
  y : Outport
  wires:
  u/1 -> Switch/3, MATLAB Function/3(u)
  robot_model/1 -> MATLAB Function/1(robot_model)
  q_fbk/1 -> Demux1/1
  Demux/1 -> MATLAB Function/4(q)
  Demux1/1 -> Demux/1
  Demux1/2 -> Terminator1/1
  Demux/2 -> Terminator/1
  Switch/1 -> y/1
  computed torque switch/1 -> Switch/2
  MATLAB Function/1(tau) -> Switch/1
  end-effector attach/1 -> MATLAB Function/2(ee_att)

== system sim_rx160_two/Robot 1 Control Algorithm/End-to-Base ==
  y : Inport  PortDimensions=6
  des : Inport  Port=2  PortDimensions=30
  fbk : Inport  Port=3  PortDimensions=30
  Constant2 : Constant  Value=ctrl_at_end
  Demux : Demux  Outputs=[12;18]
  Demux1 : Demux  Outputs=[12;18]
  Demux2 : Demux  Outputs=[12;6]
  Switch : Switch  Criteria=u2 > Threshold
  Terminator : Terminator
  Terminator1 : Terminator
  computed torque switch : Constant  Value=ctc_switch
  spatialTrnsE2B : MATLAB Function  TreatAsAtomicUnit=on
  u : Outport  PortDimensions=6
  wires:
  y/1 -> spatialTrnsE2B/5(u), Switch/3
  spatialTrnsE2B/1(y) -> Switch/1
  Constant2/1 -> Switch/2
  des/1 -> Demux/1
  Demux/1 -> spatialTrnsE2B/1(q)
  Demux/2 -> spatialTrnsE2B/2(x)
  Switch/1 -> u/1
  computed torque switch/1 -> spatialTrnsE2B/4(ctc_switch)
  fbk/1 -> Demux1/1
  Demux1/2 -> Demux2/1
  Demux2/2 -> spatialTrnsE2B/3(v)
  Demux1/1 -> Terminator/1
  Demux2/1 -> Terminator1/1

== system sim_rx160_two/Robot 1 Control Algorithm/End-to-Base Wrench ==
  y : Inport  PortDimensions=6
  des : Inport  Port=2  PortDimensions=30
  Constant2 : Constant  Value=ctrl_at_end
  Demux : Demux  Outputs=[12;18]
  Switch : Switch  Criteria=u2 > Threshold
  Terminator : Terminator
  spatialTrnsE2B : MATLAB Function  TreatAsAtomicUnit=on
  u : Outport  PortDimensions=6
  wires:
  y/1 -> Switch/3, spatialTrnsE2B/2(f_desE)
  spatialTrnsE2B/1(f_des) -> Switch/1
  Constant2/1 -> Switch/2
  des/1 -> Demux/1
  Demux/2 -> spatialTrnsE2B/1(x)
  Switch/1 -> u/1
  Demux/1 -> Terminator/1

== system sim_rx160_two/Robot 1 Control Algorithm/Error ==
  des : Inport  PortDimensions=30
  fbk : Inport  Port=2  PortDimensions=30
  Demux : Demux  Outputs=[12;18]
  Demux1 : Demux  Outputs=[12;18]
  MATLAB Function : MATLAB Function  TreatAsAtomicUnit=on
  Sum : Sum  Inputs=|+-
  Switch : Switch  Criteria=u2 > Threshold
  control_space : Constant  Value=ctrl_space
  e : Outport
  wires:
  fbk/1 -> Demux1/1
  des/1 -> Demux/1
  control_space/1 -> Switch/2
  MATLAB Function/1(y) -> Switch/1
  Demux/1 -> Sum/1
  Demux1/1 -> Sum/2
  Sum/1 -> Switch/3
  Demux/2 -> MATLAB Function/1(des)
  Demux1/2 -> MATLAB Function/2(fbk)
  Switch/1 -> e/1

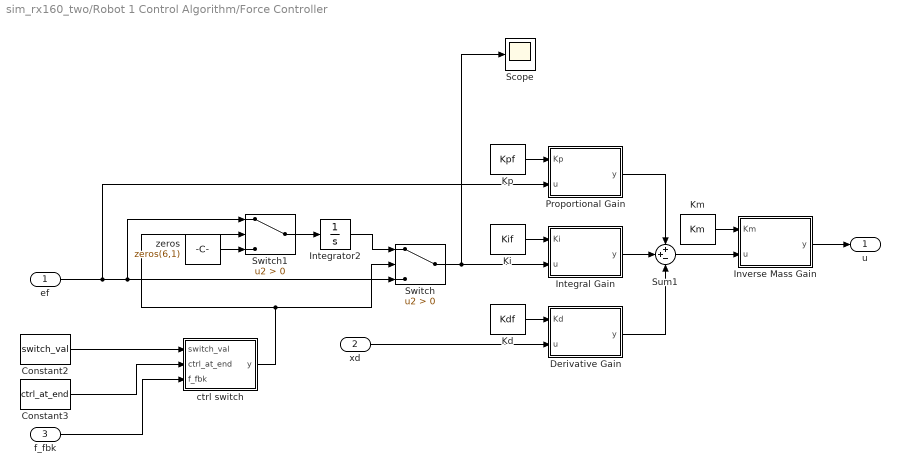
== system sim_rx160_two/Robot 1 Control Algorithm/Force Controller ==
  ef : Inport
  xd : Inport  Port=2
  f_fbk : Inport  Port=3
  Constant2 : Constant  Value=switch_val
  Constant3 : Constant  Value=ctrl_at_end
  Derivative Gain : MATLAB Function  TreatAsAtomicUnit=on
  Integral Gain : MATLAB Function  TreatAsAtomicUnit=on
  Integrator2 : Integrator
  Inverse Mass Gain : MATLAB Function  TreatAsAtomicUnit=on
  Kd : Constant  Value=Kdf
  Ki : Constant  Value=Kif
  Km : Constant  Value=Km
  Kp : Constant  Value=Kpf
  Proportional Gain : MATLAB Function  TreatAsAtomicUnit=on
  Scope : Scope
  Sum1 : Sum  Inputs=++-
  Switch : Switch  Criteria=u2 > Threshold
  Switch1 : Switch  Criteria=u2 > Threshold
  ctrl switch : MATLAB Function  TreatAsAtomicUnit=on
  zeros : Constant  Value=zeros(6,1)
  u : Outport
  wires:
  Proportional Gain/1(y) -> Sum1/1
  Integral Gain/1(y) -> Sum1/2
  ef/1 -> Switch/3, Switch1/1, Proportional Gain/2(u)
  Kp/1 -> Proportional Gain/1(Kp)
  Ki/1 -> Integral Gain/1(Ki)
  Kd/1 -> Derivative Gain/1(Kd)
  Derivative Gain/1(y) -> Sum1/3
  xd/1 -> Derivative Gain/2(u)
  Inverse Mass Gain/1(y) -> u/1
  Sum1/1 -> Inverse Mass Gain/2(u)
  Km/1 -> Inverse Mass Gain/1(Km)
  Constant3/1 -> ctrl switch/2(ctrl_at_end)
  Constant2/1 -> ctrl switch/1(switch_val)
  f_fbk/1 -> ctrl switch/3(f_fbk)
  Switch1/1 -> Integrator2/1
  Integrator2/1 -> Switch/1
  zeros/1 -> Switch1/3
  ctrl switch/1(y) -> Switch/2, Switch1/2
  Switch/1 -> Scope/1, Integral Gain/2(u)

== system sim_rx160_two/Robot 1 Control Algorithm/Kin Trns ==
  u : Inport
  q_fbk : Inport  Port=2
  Demux : Demux  Outputs=[6;6]
  Demux1 : Demux  Outputs=[12;18]
  MATLAB Function : MATLAB Function  TreatAsAtomicUnit=on
  Switch : Switch  Criteria=u2 > Threshold
  Terminator1 : Terminator
  computed torque switch : Constant  Value=ctc_switch
  control space : Constant  Value=ctrl_space
  end-effector attach : Constant  Value=ee_att_1
  robot_model : Constant  Value=robot_model_1
  y : Outport
  wires:
  u/1 -> Switch/3, MATLAB Function/4(u)
  robot_model/1 -> MATLAB Function/1(robot_model)
  Demux/1 -> MATLAB Function/5(q_pos)
  control space/1 -> Switch/2
  q_fbk/1 -> Demux1/1
  Demux1/1 -> Demux/1
  Demux/2 -> MATLAB Function/6(q_vel)
  Demux1/2 -> Terminator1/1
  Switch/1 -> y/1
  MATLAB Function/1(tau) -> Switch/1
  computed torque switch/1 -> MATLAB Function/3(ctc_switch)
  end-effector attach/1 -> MATLAB Function/2(ee_att)

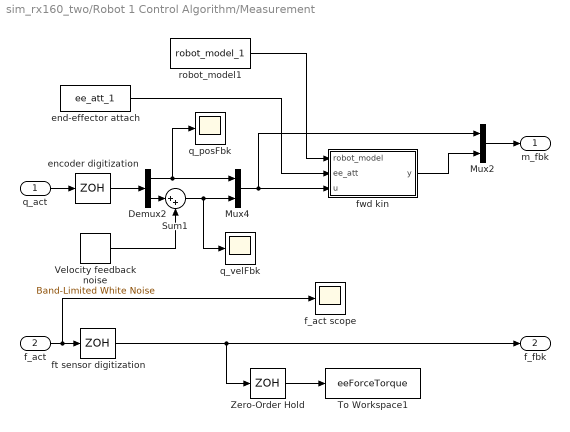
== system sim_rx160_two/Robot 1 Control Algorithm/Measurement ==
  q_act : Inport
  f_act : Inport  Port=2
  Demux2 : Demux  Outputs=2
  Mux2 : Mux  Inputs=[12;18]
  Mux4 : Mux  Inputs=2
  Sum1 : Sum  Inputs=|++
  To Workspace1 : ToWorkspace  VariableName=eeForceTorque  SaveFormat=Timeseries  SampleTime=-1
  Velocity feedback noise : simulink/Sources/Band-Limited White Noise  Cov=[0.00001]  Ts=0.01  seed=[23341]
  Zero-Order Hold : ZeroOrderHold  SampleTime=0.004
  encoder digitization : ZeroOrderHold  SampleTime=0.004
  end-effector attach : Constant  Value=ee_att_1
  f_act scope : Scope
  ft sensor digitization : ZeroOrderHold  SampleTime=0.004
  fwd kin : MATLAB Function  TreatAsAtomicUnit=on
  q_posFbk : Scope
  q_velFbk : Scope
  robot_model1 : Constant  Value=robot_model_1
  m_fbk : Outport
  f_fbk : Outport  Port=2
  wires:
  ft sensor digitization/1 -> f_fbk/1, Zero-Order Hold/1
  f_act/1 -> f_act scope/1, ft sensor digitization/1
  q_act/1 -> encoder digitization/1
  robot_model1/1 -> fwd kin/1(robot_model)
  fwd kin/1(y) -> Mux2/2
  Mux2/1 -> m_fbk/1
  Demux2/1 -> q_posFbk/1, Mux4/1
  encoder digitization/1 -> Demux2/1
  Mux4/1 -> fwd kin/3(u), Mux2/1
  Demux2/2 -> Sum1/1
  Sum1/1 -> q_velFbk/1, Mux4/2
  Velocity feedback noise/1 -> Sum1/2
  end-effector attach/1 -> fwd kin/2(ee_att)
  Zero-Order Hold/1 -> To Workspace1/1

== system sim_rx160_two/Robot 1 Control Algorithm/Motion Controller ==
  e : Inport
  Demux1 : Demux  Outputs=2
  Derivative Gain : MATLAB Function  TreatAsAtomicUnit=on
  Integral Gain : MATLAB Function  TreatAsAtomicUnit=on
  Integrator2 : Integrator
  Inverse Mass Gain : MATLAB Function  TreatAsAtomicUnit=on
  Kd : Constant  Value=Kd
  Ki : Constant  Value=Ki
  Km : Constant  Value=Km
  Kp : Constant  Value=Kp
  Proportional Gain : MATLAB Function  TreatAsAtomicUnit=on
  Scope : Scope
  Sum1 : Sum  Inputs=+++
  u : Outport
  wires:
  Derivative Gain/1(y) -> Sum1/3
  Proportional Gain/1(y) -> Sum1/1
  Integrator2/1 -> Integral Gain/2(u)
  Integral Gain/1(y) -> Sum1/2
  Demux1/2 -> Derivative Gain/2(u)
  e/1 -> Demux1/1
  Demux1/1 -> Scope/1, Proportional Gain/2(u), Integrator2/1
  Kp/1 -> Proportional Gain/1(Kp)
  Ki/1 -> Integral Gain/1(Ki)
  Kd/1 -> Derivative Gain/1(Kd)
  Km/1 -> Inverse Mass Gain/1(Km)
  Inverse Mass Gain/1(y) -> u/1
  Sum1/1 -> Inverse Mass Gain/2(u)

== system sim_rx160_two/Robot 1 Control Algorithm/Output Block ==
  m_des : Inport
  m_fbk : Inport  Port=2
  f_des : Inport  Port=3
  f_fbk : Inport  Port=4
  Demux : Demux  Outputs=2
  Demux1 : Demux  Outputs=2
  Demux2 : Demux  Outputs=[12;18]
  Demux3 : Demux  Outputs=[12;18]
  Scope : Scope  NumInputPorts=2
  Scope1 : Scope  NumInputPorts=2
  Scope2 : Scope
  Scope3 : Scope
  Terminator{,1..3} (4 alike) : Terminator
  To Workspace : ToWorkspace  VariableName=jointPosFbk  SaveFormat=Timeseries  SampleTime=-1
  To Workspace1 : ToWorkspace  VariableName=jointPosDes  SaveFormat=Timeseries  SampleTime=-1
  wires:
  Demux/2 -> Scope1/2
  Demux1/2 -> Scope1/1
  m_des/1 -> Demux2/1
  Demux2/1 -> Demux1/1
  Demux/1 -> Scope/2, To Workspace/1
  Demux1/1 -> Scope3/1, To Workspace1/1, Scope/1
  m_fbk/1 -> Demux3/1
  Demux3/1 -> Demux/1
  Demux3/2 -> Terminator/1
  Demux2/2 -> Terminator1/1
  f_des/1 -> Terminator2/1
  f_fbk/1 -> Scope2/1, Terminator3/1

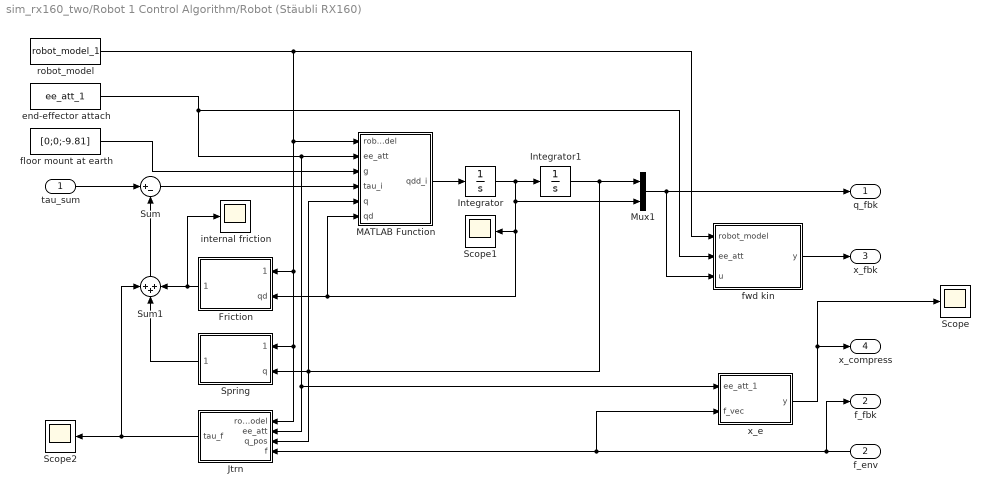
== system sim_rx160_two/Robot 1 Control Algorithm/Robot (Stäubli RX160) ==
  tau_sum : Inport
  f_env : Inport  Port=2
  Friction : MATLAB Function  TreatAsAtomicUnit=on
  Integrator : Integrator
  Integrator1 : Integrator  InitialCondition=q_posIni
  Jtrn : MATLAB Function  TreatAsAtomicUnit=on
  MATLAB Function : MATLAB Function  TreatAsAtomicUnit=on
  Mux1 : Mux  Inputs=2
  Scope : Scope
  Scope1 : Scope
  Scope2 : Scope
  Spring : MATLAB Function  TreatAsAtomicUnit=on
  Sum : Sum  Inputs=|+-
  Sum1 : Sum  Inputs=+++
  end-effector attach : Constant  Value=ee_att_1
  floor mount at earth : Constant  Value=[0;0;-9.81]
  fwd kin : MATLAB Function  TreatAsAtomicUnit=on
  internal friction : Scope
  robot_model : Constant  Value=robot_model_1
  x_e : MATLAB Function  TreatAsAtomicUnit=on
  q_fbk : Outport
  f_fbk : Outport  Port=2
  x_fbk : Outport  Port=3
  x_compress : Outport  Port=4
  wires:
  MATLAB Function/1(qdd_i) -> Integrator/1
  Sum/1 -> MATLAB Function/4(tau_i)
  Integrator1/1 -> Jtrn/3(q_pos), MATLAB Function/5(q), Spring/2(q), Mux1/1
  Integrator/1 -> MATLAB Function/6(qd), Friction/2(qd), Scope1/1, Mux1/2, Integrator1/1
  Friction/1(tau_frc) -> Sum1/3, internal friction/1
  Spring/1(tau_spr) -> Sum1/2
  robot_model/1 -> Jtrn/1(robot_model), Spring/1(robot_model), Friction/1(robot_model), MATLAB Function/1(robot_model), fwd kin/1(robot_model)
  Mux1/1 -> q_fbk/1, fwd kin/3(u)
  fwd kin/1(y) -> x_fbk/1
  Sum1/1 -> Sum/2
  tau_sum/1 -> Sum/1
  f_env/1 -> f_fbk/1, x_e/2(f_vec), Jtrn/4(f)
  Jtrn/1(tau_f) -> Sum1/1, Scope2/1
  end-effector attach/1 -> MATLAB Function/2(ee_att), Jtrn/2(ee_att), x_e/1(ee_att_1), fwd kin/2(ee_att)
  floor mount at earth/1 -> MATLAB Function/3(g)
  x_e/1(y) -> Scope/1, x_compress/1

== system sim_rx160_two/Robot 1 Control Algorithm/Selective Sum ==
  um : Inport  PortDimensions=6
  uf : Inport  Port=2  PortDimensions=6
  f_fbk : Inport  Port=3  PortDimensions=6
  Constant : Constant  Value=Sx_diag
  Constant1 : Constant  Value=Sf_diag
  Constant2 : Constant  Value=switch_val
  Constant3 : Constant  Value=ctrl_at_end
  MATLAB Function : MATLAB Function  TreatAsAtomicUnit=on
  Out1 : Outport  PortDimensions=6
  wires:
  uf/1 -> MATLAB Function/6(uf)
  um/1 -> MATLAB Function/1(um)
  MATLAB Function/1(y) -> Out1/1
  Constant/1 -> MATLAB Function/2(Sx_diag)
  Constant1/1 -> MATLAB Function/5(Sf_diag)
  Constant2/1 -> MATLAB Function/3(switch_val)
  f_fbk/1 -> MATLAB Function/7(f_fbk)
  Constant3/1 -> MATLAB Function/4(ctrl_at_end)

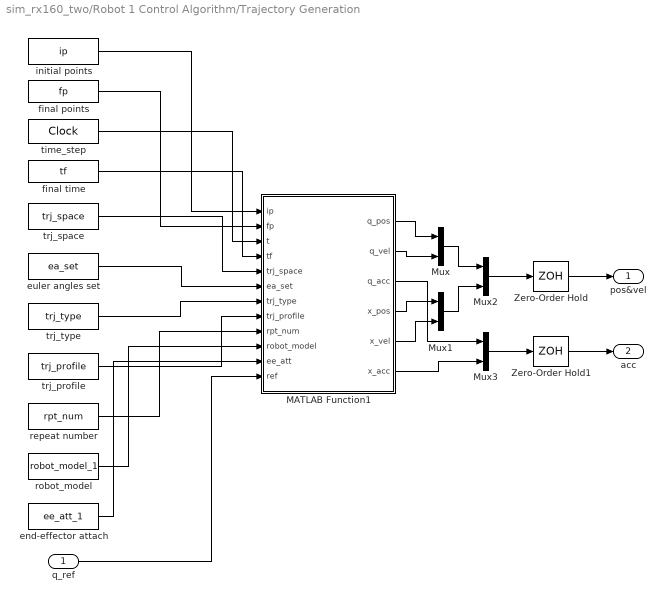
== system sim_rx160_two/Robot 1 Control Algorithm/Trajectory Generation ==
  q_ref : Inport
  MATLAB Function1 : MATLAB Function  TreatAsAtomicUnit=on
  Mux{,1..3} (4 alike) : Mux  Inputs=2
  Zero-Order Hold : ZeroOrderHold  SampleTime=0.004
  Zero-Order Hold1 : ZeroOrderHold  SampleTime=0.004
  end-effector attach : Constant  Value=ee_att_1
  euler angles set : Constant  Value=ea_set
  final points : Constant  Value=fp
  final time : Constant  Value=tf
  initial points : Constant  Value=ip
  repeat number : Constant  Value=rpt_num
  robot_model : Constant  Value=robot_model_1
  time_step : DigitalClock  SampleTime=0.004
  trj_profile : Constant  Value=trj_profile
  trj_space : Constant  Value=trj_space
  trj_type : Constant  Value=trj_type
  pos&vel : Outport
  acc : Outport  Port=2
  wires:
  trj_profile/1 -> MATLAB Function1/8(trj_profile)
  MATLAB Function1/1(q_pos) -> Mux/1
  time_step/1 -> MATLAB Function1/3(t)
  robot_model/1 -> MATLAB Function1/10(robot_model)
  initial points/1 -> MATLAB Function1/1(ip)
  final time/1 -> MATLAB Function1/4(tf)
  final points/1 -> MATLAB Function1/2(fp)
  MATLAB Function1/2(q_vel) -> Mux/2
  trj_space/1 -> MATLAB Function1/5(trj_space)
  MATLAB Function1/5(x_vel) -> Mux1/2
  MATLAB Function1/4(x_pos) -> Mux1/1
  Mux2/1 -> Zero-Order Hold/1
  Mux1/1 -> Mux2/2
  Mux/1 -> Mux2/1
  q_ref/1 -> MATLAB Function1/12(ref)
  Zero-Order Hold/1 -> pos&vel/1
  MATLAB Function1/3(q_acc) -> Mux3/1
  MATLAB Function1/6(x_acc) -> Mux3/2
  Mux3/1 -> Zero-Order Hold1/1
  euler angles set/1 -> MATLAB Function1/6(ea_set)
  Zero-Order Hold1/1 -> acc/1
  trj_type/1 -> MATLAB Function1/7(trj_type)
  end-effector attach/1 -> MATLAB Function1/11(ee_att)
  repeat number/1 -> MATLAB Function1/9(rpt_num)
